simulink library "furuta_lib"  (Simulink 4.00)
values from neighbouring files (symbols this model uses):
  Fscomp_neg = 0.01    [furuta_init.m]
  Fscomp_pos = 0.01    [furuta_init.m]
  g = 9.81    [furuta_init.m]
  h = 0.01    [furuta_init.m]
  Jarm = ma*g*r_cm/wa^2    (= 0.00140535509218)    [furuta_init.m]
  Jm = 0.0000381    (= 3.81e-05)    [furuta_init.m]
  lp = 0.421    [furuta_init.m]
  M = 0.015    [furuta_init.m]
  ma = 0.165    [furuta_init.m]
  mpa = 0.02    [furuta_init.m]
  r = 0.245    [furuta_init.m]
  x0 = x_0    [furuta.m]    (also in furuta_init.m = [0.1 0 0 0]')
settings Model: Creator=jakesson  LastModifiedBy=jakesson  ExtModeAutoUpdateStatusClock=off

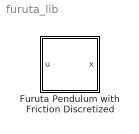
== system furuta_lib ==
  Furuta Pendulum with Friction Discretized : Subsystem  AncestorBlock=|
      | furuta_lib/Furuta Pendulum
      | with Friction
      | Discretized
      settings: RTWFcnNameOpts=Auto  RTWFileNameOpts=Auto

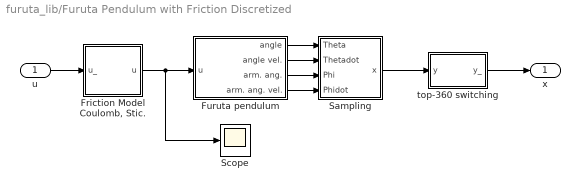
== system furuta_lib/Furuta Pendulum with Friction Discretized ==
  u : Inport  Port=1  LatchInput=off
  "Friction Model Coulomb, Stic." : Subsystem
      settings: RTWFcnNameOpts=Auto  RTWFileNameOpts=Auto
  Furuta pendulum : Subsystem  mask{lp=lp, M=M, mpa=mpa, r=r, ma=ma, Jarm=Jarm, Jm=Jm, g=g, x_0=x0}
      mask prompts: lp "Pendulum Length"; M "Mass of Pendulum weight"; mpa "Mass of pendulum without weight"; r "Length of Arm"; ma "Mass of Arm"; Jarm "Moment of inertia of Arm"; Jm "Moment of inertia of Motor"
      settings: RTWFcnNameOpts=Auto  RTWFileNameOpts=Auto
  Sampling : Subsystem
      settings: RTWFcnNameOpts=Auto  RTWFileNameOpts=Auto
  Scope : Scope
      settings: TimeRange=auto  YMin=-5  YMax=5  SaveToWorkspace=off  MaxDataPoints=5000
  top-360 switching : Subsystem
      settings: RTWFcnNameOpts=Auto  RTWFileNameOpts=Auto
  x : Outport  Port=1  InitialOutput=0
  wires:
  "Friction Model Coulomb, Stic."/1(u) -> Scope/1, Furuta pendulum/1(u)
  top-360 switching/1(y_) -> x/1
  Sampling/1(x) -> top-360 switching/1(y)
  u/1 -> "Friction Model Coulomb, Stic."/1(u_)
  Furuta pendulum/2(angle vel.) -> Sampling/2(Thetadot)
  Furuta pendulum/3(arm. ang.) -> Sampling/3(Phi)
  Furuta pendulum/4(arm. ang. vel.) -> Sampling/4(Phidot)
  Furuta pendulum/1(angle) -> Sampling/1(Theta)

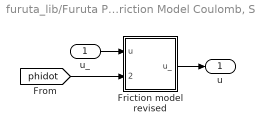
== system furuta_lib/Furuta Pendulum with Friction Discretized/Friction Model Coulomb, Stic. ==
  u_ : Inport  Port=1  LatchInput=off
  Friction model revised : Subsystem
      settings: RTWFcnNameOpts=Auto  RTWFileNameOpts=Auto
  u : Outport  Port=1  InitialOutput=0
  wires:
  Friction model revised/1(u_) -> u/1
  [phidot] -> Friction model revised/2(phidot)
  u_/1 -> Friction model revised/1(u)

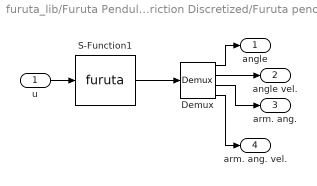
== system furuta_lib/Furuta Pendulum with Friction Discretized/Furuta pendulum ==
  u : Inport  Port=1  LatchInput=off
  Demux : Demux  Outputs=4  BusSelectionMode=off
  S-Function1 : S-Function  FunctionName=furuta  Parameters=lp,M,mpa,r,ma,Jarm,Jm,g,x_0  PortCounts=[]  SFunctionModules=''
  angle : Outport  Port=1  InitialOutput=0
  angle vel. : Outport  Port=2  InitialOutput=0
  arm. ang. : Outport  Port=3  InitialOutput=0
  arm. ang. vel. : Outport  Port=4  InitialOutput=0
  wires:
  Demux/4 -> arm. ang. vel./1
  Demux/3 -> arm. ang./1
  u/1 -> S-Function1/1
  Demux/2 -> angle vel./1
  Demux/1 -> angle/1
  S-Function1/1 -> Demux/1

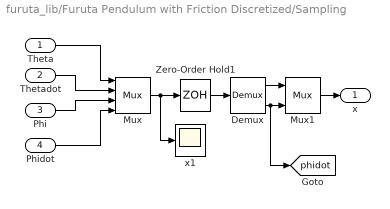
== system furuta_lib/Furuta Pendulum with Friction Discretized/Sampling ==
  Theta : Inport  Port=1  LatchInput=off
  Thetadot : Inport  Port=2  LatchInput=off
  Phi : Inport  Port=3  LatchInput=off
  Phidot : Inport  Port=4  LatchInput=off
  Demux : Demux  Outputs=[3 1]  BusSelectionMode=off
  Mux : Mux  Inputs=4
      settings: DisplayOption=none
  Mux1 : Mux  Inputs=2
      settings: DisplayOption=none
  Zero-Order Hold1 : ZeroOrderHold  SampleTime=h
  x1 : Scope
      settings: TimeRange=auto  YMin=-1.5  YMax=2.5  SaveToWorkspace=off  MaxDataPoints=5000
  x : Outport  Port=1  InitialOutput=0
  tag scope: phidot=global
  wires:
  Zero-Order Hold1/1 -> Demux/1
  Mux/1 -> Zero-Order Hold1/1, x1/1
  Demux/1 -> Mux1/1
  Mux1/1 -> x/1
  Phi/1 -> Mux/3
  Thetadot/1 -> Mux/2
  Theta/1 -> Mux/1
  Phidot/1 -> Mux/4
  Demux/2 -> Mux1/2, [phidot]

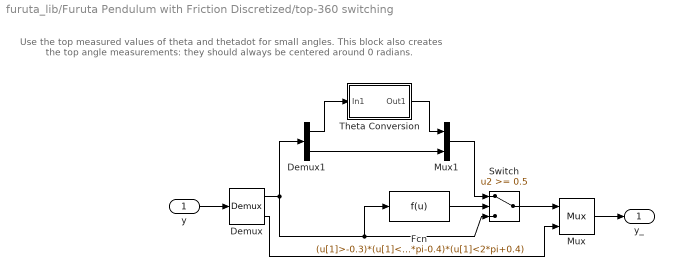
== system furuta_lib/Furuta Pendulum with Friction Discretized/top-360 switching ==
  note: Use the top measured values of
      | theta and thetadot for small angles.
      | This block also creates the top angle
      | measurements: they should always be
      | centered around 0 radians.
  y : Inport  Port=1  LatchInput=off
  Demux : Demux  Outputs=[2 2]  BusSelectionMode=off
  Demux1 : Demux  Outputs=2  BusSelectionMode=off
  Fcn : Fcn  Expr=(u[1]>-0.3)*(u[1]<0.4)+(u[1]>2*pi-0.4)*(u[1]<2*pi+0.4)
  Mux : Mux  Inputs=2
      settings: DisplayOption=none
  Mux1 : Mux  Inputs=2
  Switch : Switch  Threshold=0.5
  Theta Conversion : Subsystem
      settings: RTWFcnNameOpts=Auto  RTWFileNameOpts=Auto
  y_ : Outport  Port=1
  wires:
  Fcn/1 -> Switch/2
  Switch/1 -> Mux/1
  Mux/1 -> y_/1
  y/1 -> Demux/1
  Demux/2 -> Mux/2
  Demux/1 -> Demux1/1, Switch/3, Fcn/1
  Demux1/1 -> Theta Conversion/1(In1)
  Theta Conversion/1(Out1) -> Mux1/1
  Demux1/2 -> Mux1/2
  Mux1/1 -> Switch/1

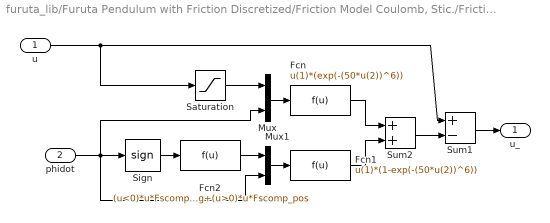
== system furuta_lib/Furuta Pendulum with Friction Discretized/Friction Model Coulomb, Stic./Friction model revised ==
  u : Inport  Port=1  LatchInput=off
  phidot : Inport  Port=2  LatchInput=off
  Fcn : Fcn  Expr=u(1)*(exp(-(50*u(2))^6))
  Fcn1 : Fcn  Expr=u(1)*(1-exp(-(50*u(2))^6))
  Fcn2 : Fcn  Expr=(u<0)*u*Fscomp_neg+(u>0)*u*Fscomp_pos
  Mux : Mux  Inputs=2
  Mux1 : Mux  Inputs=2
  Saturation : Saturate  UpperLimit=Fscomp_pos  LowerLimit=-Fscomp_neg  LinearizeAsGain=on
  Sign : Signum
  Sum1 : Sum  Inputs=+-  SaturateOnIntegerOverflow=on
  Sum2 : Sum  Inputs=++  SaturateOnIntegerOverflow=on
  u_ : Outport  Port=1  InitialOutput=0
  wires:
  Fcn2/1 -> Mux1/1
  Sign/1 -> Fcn2/1
  Fcn1/1 -> Sum2/2
  Mux1/1 -> Fcn1/1
  Saturation/1 -> Mux/1
  Mux/1 -> Fcn/1
  Fcn/1 -> Sum2/1
  phidot/1 -> Mux/2, Mux1/2, Sign/1
  Sum1/1 -> u_/1
  u/1 -> Saturation/1, Sum1/1
  Sum2/1 -> Sum1/2

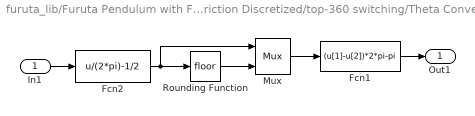
== system furuta_lib/Furuta Pendulum with Friction Discretized/top-360 switching/Theta Conversion ==
  In1 : Inport  Port=1  LatchInput=off
  Fcn1 : Fcn  Expr=(u[1]-u[2])*2*pi-pi
  Fcn2 : Fcn  Expr=u/(2*pi)-1/2
  Mux : Mux  Inputs=2
      settings: DisplayOption=none
  Rounding Function : Rounding  Operator=floor
  Out1 : Outport  Port=1  InitialOutput=0
  wires:
  In1/1 -> Fcn2/1
  Fcn1/1 -> Out1/1
  Mux/1 -> Fcn1/1
  Fcn2/1 -> Mux/1, Rounding Function/1
  Rounding Function/1 -> Mux/2
